simulink model "SVPWM_32bianhuan_"  (Simulink 7.6)
settings: Solver=ode45  StartTime=0.0  StopTime=0.5  FixedStep=1e-7  MaxStep=1e-5  MinStep=1e-6  RelTol=1e-3
libraries: powerlib x23, powerlib_extras x5, simulink x1
settings Model: Creator=Administrator  LastModifiedBy=huanglei
settings OptimizationCC: InitFltsAndDblsToZero=on
settings DebuggingCC: AlgebraicLoopMsg=none  SaveWithParameterizedLinksMsg=none  SignalResolutionControl=TryResolveAllWithWarning  MultiTaskDSMMsg=warning  MultiTaskCondExecSysMsg=none  StrictBusMsg=None
settings RTWCC: IncludeERTFirstTime=on
settings GRTTargetCC: TargetFcnLib=ansi_tfl_tmw.mat

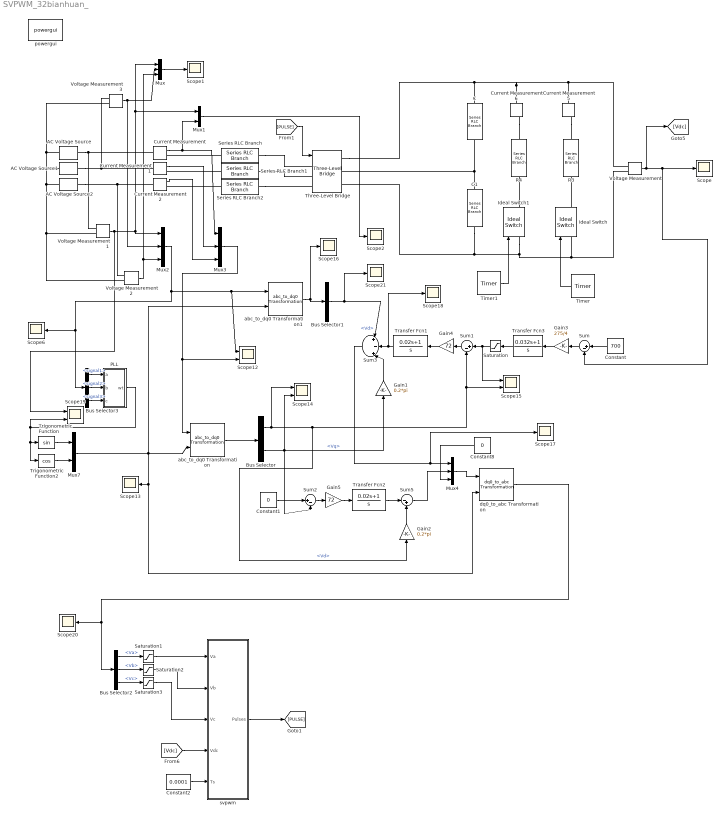
== system SVPWM_32bianhuan_ ==
  AC Voltage Source : powerlib/Electrical Sources/AC Voltage Source  DialogController=POWERSYS.PowerSysDialog  SystemSampleTime=-1  Amplitude=311  Phase=90  Frequency=50  SampleTime=0  Measurements=None
  AC Voltage Source1 : powerlib/Electrical Sources/AC Voltage Source  DialogController=POWERSYS.PowerSysDialog  SystemSampleTime=-1  Amplitude=311  Phase=-30  Frequency=50  SampleTime=0  Measurements=None
  AC Voltage Source2 : powerlib/Electrical Sources/AC Voltage Source  DialogController=POWERSYS.PowerSysDialog  SystemSampleTime=-1  Amplitude=311  Phase=210  Frequency=50  SampleTime=0  Measurements=None
  Bus Selector : BusSelector  OutputSignals=Vd,Vq
  Bus Selector1 : BusSelector  OutputSignals=Vd
  Bus Selector2 : BusSelector  OutputSignals=Va,Vb,Vc
  Bus Selector3 : BusSelector  OutputSignals=signal1,signal2,signal3
  C : powerlib/Elements/Series RLC Branch  DialogController=POWERSYS.PowerSysDialog  PhysicalDomain=powersysdomain  SubClassName=unknown  LeftPortType=p1  RightPortType=p1  LConnTagsString=__new0  RConnTagsString=__new0  BranchType=C  Resistance=1  Inductance=1e-3  SetiL0=off  InitialCurrent=0  Capacitance=1e-3  Setx0=off  InitialVoltage=0  Measurements=None
  C1 : powerlib/Elements/Series RLC Branch  DialogController=POWERSYS.PowerSysDialog  PhysicalDomain=powersysdomain  SubClassName=unknown  LeftPortType=p1  RightPortType=p1  LConnTagsString=__new0  RConnTagsString=__new0  BranchType=C  Resistance=1  Inductance=1e-3  SetiL0=off  InitialCurrent=0  Capacitance=1e-3  Setx0=off  InitialVoltage=0  Measurements=None
  Constant : Constant  Value=700
  Constant1 : Constant  Value=0
  Constant2 : Constant  Value=0.0001
  Constant8 : Constant  Value=0
  Current Measurement{,1..2,5..6} (5 alike) : powerlib/Measurements/Current Measurement  DialogController=POWERSYS.PowerSysDialog  SystemSampleTime=-1  PhasorSimulation=off  OutputType=Complex  PSBequivalent=0
  Gain1 : Gain  Gain=0.2*pi
  Gain2 : Gain  Gain=0.2*pi
  Gain3 : Gain  Gain=275/4
  Gain4 : Gain  Gain=72
  Gain5 : Gain  Gain=72
  Ideal Switch : powerlib/Power Electronics/Ideal Switch  DialogController=POWERSYS.PowerSysDialog  SystemSampleTime=-1  Ron=0.001  Lon=0  IC=0  Rs=1e5  Cs=inf  Measurements=on
  Ideal Switch1 : powerlib/Power Electronics/Ideal Switch  DialogController=POWERSYS.PowerSysDialog  SystemSampleTime=-1  Ron=0.001  Lon=0  IC=0  Rs=1e5  Cs=inf  Measurements=on
  Mux{,2..4} (4 alike) : Mux  Inputs=3
  Mux1 : Mux  Inputs=2
  Mux7 : Mux  Inputs=2
  PLL : Subsystem
  R3 : powerlib/Elements/Series RLC Branch  DialogController=POWERSYS.PowerSysDialog  PhysicalDomain=powersysdomain  SubClassName=unknown  LeftPortType=p1  RightPortType=p1  LConnTagsString=__new0  RConnTagsString=__new0  BranchType=R  Resistance=100  Inductance=1e-3  SetiL0=off  InitialCurrent=0  Capacitance=1e-6  Setx0=off  InitialVoltage=0  Measurements=None
  R4 : powerlib/Elements/Series RLC Branch  DialogController=POWERSYS.PowerSysDialog  PhysicalDomain=powersysdomain  SubClassName=unknown  LeftPortType=p1  RightPortType=p1  LConnTagsString=__new0  RConnTagsString=__new0  BranchType=R  Resistance=50  Inductance=1e-3  SetiL0=off  InitialCurrent=0  Capacitance=1e-6  Setx0=off  InitialVoltage=0  Measurements=None
  Saturation : Saturate  UpperLimit=200  LowerLimit=-200
  Saturation1 : Saturate  UpperLimit=220  LowerLimit=-220
  Saturation2 : Saturate  UpperLimit=220  LowerLimit=-220
  Saturation3 : Saturate  UpperLimit=220  LowerLimit=-220
  Scope{,1..2,6,13,16..18,20..21} (10 alike) : Scope
      Scope settings: TimeRange=0.5  YMin=698.5  YMax=707
      Scope1 settings: YMin=-400  YMax=400
      Scope13 settings: YMin=-1  YMax=0.6  SaveName=ScopeData13
      Scope16 settings: YMin=-25  YMax=325  SaveName=ScopeData16
      Scope17 settings: YMin=21050  YMax=22150  SaveName=ScopeData17
      Scope18 settings: YMin=-20775  YMax=-20425  SaveName=ScopeData18
      Scope2 settings: YMin=-350  YMax=350  SaveName=ScopeData2
      Scope20 settings: YMin=-1  YMax=1  SaveName=ScopeData20
      Scope21 settings: YMin=311  YMax=311  SaveName=ScopeData21
      Scope6 settings: YMin=-400  YMax=400  SaveName=ScopeData6
  Scope{12,14..15,19} (4 alike) : Scope  NumInputPorts=2
      Scope12 settings: YMin=-4~-5  YMax=4~5  SaveName=ScopeData12
      Scope14 settings: YMin=15~-2.25  YMax=26~3.25  SaveName=ScopeData14
      Scope15 settings: YMin=-503.7~-1  YMax=-503.425~1  SaveName=ScopeData15
      Scope19 settings: YMin=0~-5  YMax=6.5~5  SaveName=ScopeData19
  Series RLC Branch : powerlib/Elements/Series RLC Branch  DialogController=POWERSYS.PowerSysDialog  PhysicalDomain=powersysdomain  SubClassName=unknown  LeftPortType=p1  RightPortType=p1  LConnTagsString=__new0  RConnTagsString=__new0  BranchType=RL  Resistance=0.1  Inductance=2e-3  SetiL0=off  InitialCurrent=0  Capacitance=1e-6  Setx0=off  InitialVoltage=0  Measurements=None
  Series RLC Branch1 : powerlib/Elements/Series RLC Branch  DialogController=POWERSYS.PowerSysDialog  PhysicalDomain=powersysdomain  SubClassName=unknown  LeftPortType=p1  RightPortType=p1  LConnTagsString=__new0  RConnTagsString=__new0  BranchType=RL  Resistance=0.1  Inductance=2e-3  SetiL0=off  InitialCurrent=0  Capacitance=1e-6  Setx0=off  InitialVoltage=0  Measurements=None
  Series RLC Branch2 : powerlib/Elements/Series RLC Branch  DialogController=POWERSYS.PowerSysDialog  PhysicalDomain=powersysdomain  SubClassName=unknown  LeftPortType=p1  RightPortType=p1  LConnTagsString=__new0  RConnTagsString=__new0  BranchType=RL  Resistance=0.1  Inductance=2e-3  SetiL0=off  InitialCurrent=0  Capacitance=1e-6  Setx0=off  InitialVoltage=0  Measurements=None
  Sum : Sum  Inputs=|+-
  Sum1 : Sum  Inputs=|+-
  Sum2 : Sum  Inputs=|+-
  Sum3 : Sum  Inputs=|+|-|+|
  Sum5 : Sum  Inputs=|-+
  Three-Level Bridge : powerlib/Power Electronics/Three-Level Bridge  DialogController=POWERSYS.PowerSysDialog  SystemSampleTime=-1  Arms=3  SnubberResistance=1e5  SbubberCapacitance=inf  Device=IGBT / Diodes  Ron=1e-3  ForwardVoltages="[  0  0  ]"  Measurements=None
  Timer : powerlib_extras/Control  Blocks/Timer  DialogController=POWERSYS.PowerSysDialog  SystemSampleTime=-1  t=[0 0.3]  e=[0 1]
  Timer1 : powerlib_extras/Control  Blocks/Timer  DialogController=POWERSYS.PowerSysDialog  SystemSampleTime=-1  t=[0 0.3]  e=[1 0]
  Transfer Fcn1 : TransferFcn  Numerator=[0.02 1]  Denominator=[1 0]
  Transfer Fcn2 : TransferFcn  Numerator=[0.02 1]  Denominator=[1 0]
  Transfer Fcn3 : TransferFcn  Numerator=[0.032 1]  Denominator=[1 0]
  Trigonometric Function : Trigonometry
  Trigonometric Function2 : Trigonometry  Operator=cos
  Voltage Measurement{,1..3} (4 alike) : powerlib/Measurements/Voltage Measurement  DialogController=POWERSYS.PowerSysDialog  SystemSampleTime=-1  PhasorSimulation=off  OutputType=Complex  PSBequivalent=0
  abc_to_dq0 Transformation : powerlib_extras/Measurements/abc_to_dq0 Transformation  DialogController=POWERSYS.PowerSysDialog  SystemSampleTime=-1
  abc_to_dq0 Transformation1 : powerlib_extras/Measurements/abc_to_dq0 Transformation  DialogController=POWERSYS.PowerSysDialog  SystemSampleTime=-1
  dq0_to_abc Transformation : powerlib_extras/Measurements/dq0_to_abc Transformation  DialogController=POWERSYS.PowerSysDialog  SystemSampleTime=-1
  powergui : powerlib/powergui  Priority=1  SystemSampleTime=-1  SimulationMode=Discrete  SampleTime=50e-6  frequency=60  SPID=off  DisableSnubberDevices=off  DisableRonSwitches=off  DisableVfSwitches=off  SwTol=0  Interpol=off  frequencyindice=50  echomessages=off  HookPort=off  DisplayEquations=off  FunctionMessages=off  EnableUseOfTLC=off  x0status=blocks  RestoreLinks=warning  ResistiveCurrentMeasurement=off  Frange=[0:2:500]  Ylog=off  Xlog=on  ShowGrid=off  save=off  variable=ZData  ZoomFFT=off  StartTime=0.0  cycles=1  DisplayStyle=1  fundamental=60  FreqAxis=off  MaxFrequency=1000  frequencyindicesteady=1  RmsSteady=1  display=off  Ts=0  methode=off
  svpwm : Subsystem
  wires:
  Voltage Measurement/1 -> Scope/1, Sum/2, [Vdc]
  Current Measurement/1 -> Mux1/2, Mux3/1
  Voltage Measurement1/1 -> Scope19/1, Mux2/1, Mux/1, Mux1/1
  Voltage Measurement3/1 -> Mux/2, Mux2/2
  Mux/1 -> Scope1/1
  Mux1/1 -> Scope2/1
  Voltage Measurement2/1 -> Mux/3, Mux2/3
  Constant/1 -> Sum/1
  Mux2/1 -> Scope6/1, Bus Selector3/1, Scope12/1, abc_to_dq0 Transformation1/1
  Current Measurement1/1 -> Mux3/2
  Current Measurement2/1 -> Mux3/3
  Mux3/1 -> abc_to_dq0 Transformation/1, Scope12/2
  abc_to_dq0 Transformation/1 -> Bus Selector/1
  Bus Selector/1 -> Gain2/1, Sum1/2, Scope15/2, Scope14/1  "<Vd>"
  Sum1/1 -> Gain4/1
  Constant1/1 -> Sum2/1
  Bus Selector/2 -> Scope14/2, Gain1/1, Sum2/2  "<Vq>"
  Sum2/1 -> Gain5/1
  Gain1/1 -> Sum3/3
  Gain2/1 -> Sum5/2
  abc_to_dq0 Transformation1/1 -> Bus Selector1/1, Scope16/1
  Bus Selector1/1 -> Sum3/1, Scope21/1  "<Vd>"
  Sum3/1 -> Mux4/1, Scope17/1
  Sum5/1 -> Mux4/2
  Mux4/1 -> dq0_to_abc Transformation/1
  dq0_to_abc Transformation/1 -> Bus Selector2/1, Scope20/1
  Constant8/1 -> Mux4/3
  Trigonometric Function2/1 -> Mux7/2
  Trigonometric Function/1 -> Mux7/1
  Bus Selector3/1 -> PLL/1(a)  "<signal1>"
  Bus Selector3/2 -> PLL/2(b)  "<signal2>"
  Bus Selector3/3 -> PLL/3(c)  "<signal3>"
  Mux7/1 -> abc_to_dq0 Transformation1/2, abc_to_dq0 Transformation/2, Scope13/1, dq0_to_abc Transformation/2
  PLL/1(wt) -> Trigonometric Function/1, Trigonometric Function2/1, Scope19/2
  Sum/1 -> Gain3/1
  Gain3/1 -> Transfer Fcn3/1
  Gain4/1 -> Transfer Fcn1/1
  Gain5/1 -> Transfer Fcn2/1
  Transfer Fcn3/1 -> Saturation/1
  Transfer Fcn2/1 -> Sum5/1
  Transfer Fcn1/1 -> Sum3/2, Scope18/1
  Saturation/1 -> Scope15/1, Sum1/1
  Timer/1 -> Ideal Switch/1
  Timer1/1 -> Ideal Switch1/1
  Constant2/1 -> svpwm/5(Ts)
  [Vdc] -> svpwm/4(Vdc)
  svpwm/1(Pulses) -> [PULSE]
  [PULSE] -> Three-Level Bridge/1
  Bus Selector2/1 -> Saturation1/1  "<Va>"
  Saturation1/1 -> svpwm/1(Va)
  Bus Selector2/2 -> Saturation2/1  "<Vb>"
  Bus Selector2/3 -> Saturation3/1  "<Vc>"
  Saturation2/1 -> svpwm/2(Vb)
  Saturation3/1 -> svpwm/3(Vc)
  connections:
  AC Voltage Source/RConn1 -- Current Measurement/LConn1 -- Voltage Measurement1/LConn1
  AC Voltage Source1/RConn1 -- Current Measurement1/LConn1 -- Voltage Measurement3/LConn1
  AC Voltage Source2/RConn1 -- Current Measurement2/LConn1 -- Voltage Measurement2/LConn1
  Voltage Measurement3/LConn2 -- Voltage Measurement1/LConn2 -- Voltage Measurement2/LConn2 -- AC Voltage Source2/LConn1 -- AC Voltage Source1/LConn1 -- AC Voltage Source/LConn1
  Series RLC Branch/LConn1 -- Current Measurement/RConn1
  Series RLC Branch1/LConn1 -- Current Measurement1/RConn1
  Series RLC Branch2/LConn1 -- Current Measurement2/RConn1
  Current Measurement5/RConn1 -- R3/RConn1
  Ideal Switch/RConn1 -- R3/LConn1
  Current Measurement6/RConn1 -- R4/RConn1
  Ideal Switch1/RConn1 -- R4/LConn1
  Series RLC Branch/RConn1 -- Three-Level Bridge/LConn1
  Series RLC Branch1/RConn1 -- Three-Level Bridge/LConn2
  Series RLC Branch2/RConn1 -- Three-Level Bridge/LConn3
  C1/LConn1 -- C/RConn1 -- Three-Level Bridge/RConn2
  Three-Level Bridge/RConn1 -- C/LConn1 -- Current Measurement6/LConn1 -- Voltage Measurement/LConn1 -- Current Measurement5/LConn1
  C1/RConn1 -- Three-Level Bridge/RConn3 -- Ideal Switch1/LConn1 -- Voltage Measurement/LConn2 -- Ideal Switch/LConn1

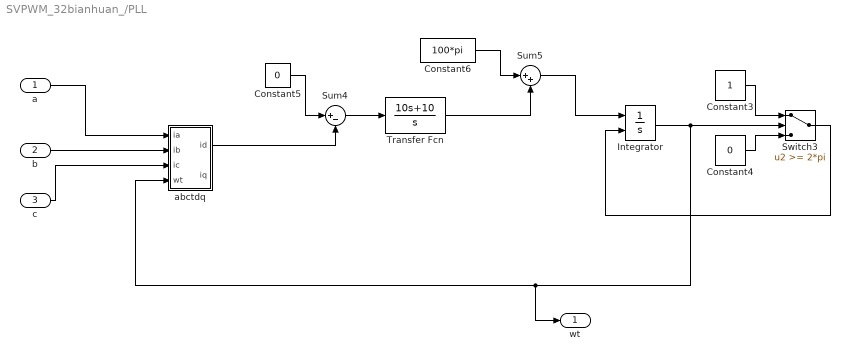
== system SVPWM_32bianhuan_/PLL ==
  a : Inport
  b : Inport  Port=2
  c : Inport  Port=3
  Constant3 : Constant
  Constant4 : Constant  Value=0
  Constant5 : Constant  Value=0
  Constant6 : Constant  Value=100*pi
  Integrator : Integrator  ExternalReset=rising
  Sum4 : Sum  Inputs=|+-
  Sum5 : Sum  Inputs=|++
  Switch3 : Switch  Threshold=2*pi
  Transfer Fcn : TransferFcn  Numerator=[10 10]  Denominator=[1 0]
  abctdq : Subsystem
  wt : Outport
  wires:
  Constant3/1 -> Switch3/1
  Switch3/1 -> Integrator/2
  Constant4/1 -> Switch3/3
  Integrator/1 -> Switch3/2, wt/1, abctdq/4(wt)
  a/1 -> abctdq/1(ia)
  Constant5/1 -> Sum4/1
  abctdq/1(id) -> Sum4/2
  b/1 -> abctdq/2(ib)
  c/1 -> abctdq/3(ic)
  Constant6/1 -> Sum5/1
  Sum5/1 -> Integrator/1
  Transfer Fcn/1 -> Sum5/2
  Sum4/1 -> Transfer Fcn/1

== system SVPWM_32bianhuan_/svpwm ==
  Va : Inport
  Vb : Inport  Port=2
  Vc : Inport  Port=3
  Vdc : Inport  Port=4
  Ts : Inport  Port=5
  Repeating Sequence1 : simulink/Sources/Repeating Sequence  SystemSampleTime=-1  rep_seq_t=[0 0.00005 0.0001]  rep_seq_y=[0 0.00005 0]
  Scope : Scope
      settings: SaveName=ScopeData7
  Sub4 abc__alpha_beta : Subsystem
  Subsystem5 : Subsystem
  Pulses : Outport
  wires:
  Vc/1 -> Sub4 abc__alpha_beta/3(Vc)
  Sub4 abc__alpha_beta/2(Vbeta) -> Subsystem5/2(Vbeta)
  Sub4 abc__alpha_beta/1(Valfa) -> Subsystem5/1(Valfa), Scope/1
  Vb/1 -> Sub4 abc__alpha_beta/2(Vb)
  Va/1 -> Sub4 abc__alpha_beta/1(Va)
  Subsystem5/1(Pulses) -> Pulses/1
  Vdc/1 -> Subsystem5/3(Vdc)
  Ts/1 -> Subsystem5/4(Ts)
  Repeating Sequence1/1 -> Subsystem5/5(wave)

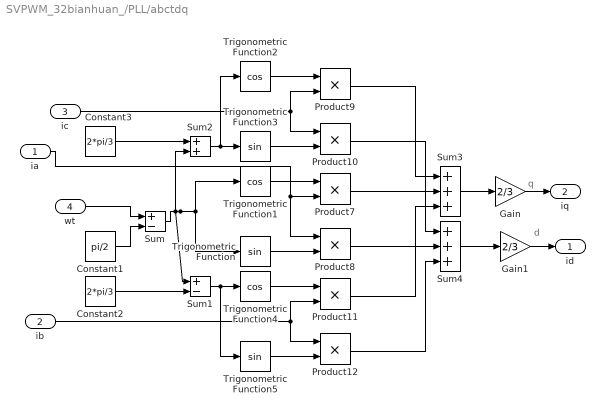
== system SVPWM_32bianhuan_/PLL/abctdq ==
  note: d
  note: q
  ia : Inport
  ib : Inport  Port=2
  ic : Inport  Port=3
  wt : Inport  Port=4
  Constant1 : Constant  Value=pi/2
  Constant2 : Constant  Value=2*pi/3
  Constant3 : Constant  Value=2*pi/3
  Gain : Gain  Gain=2/3
  Gain1 : Gain  Gain=2/3
  Product{7..12} (6 alike) : Product  RndMeth=Zero
  Sum : Sum  Inputs=+-
  Sum1 : Sum  Inputs=+-
  Sum2 : Sum
  Sum3 : Sum  Inputs=+++
  Sum4 : Sum  Inputs=+++
  Trigonometric Function : Trigonometry
  Trigonometric Function1 : Trigonometry  Operator=cos
  Trigonometric Function2 : Trigonometry  Operator=cos
  Trigonometric Function3 : Trigonometry
  Trigonometric Function4 : Trigonometry  Operator=cos
  Trigonometric Function5 : Trigonometry
  id : Outport
  iq : Outport  Port=2
  wires:
  ic/1 -> Product10/1, Product9/2
  ia/1 -> Product8/1, Product7/2
  ib/1 -> Product12/1, Product11/2
  Sum4/1 -> Gain1/1
  Sum3/1 -> Gain/1
  Product11/1 -> Sum3/3
  Product9/1 -> Sum3/1
  Product10/1 -> Sum4/1
  Product12/1 -> Sum4/3
  Product7/1 -> Sum3/2
  Product8/1 -> Sum4/2
  Trigonometric Function5/1 -> Product12/2
  Trigonometric Function4/1 -> Product11/1
  Trigonometric Function/1 -> Product8/2
  Trigonometric Function1/1 -> Product7/1
  Trigonometric Function3/1 -> Product10/2
  Trigonometric Function2/1 -> Product9/1
  Sum1/1 -> Trigonometric Function4/1, Trigonometric Function5/1
  Constant1/1 -> Sum/2
  Sum2/1 -> Trigonometric Function2/1, Trigonometric Function3/1
  Constant3/1 -> Sum2/1
  Constant2/1 -> Sum1/2
  Sum/1 -> Trigonometric Function/1, Trigonometric Function1/1, Sum1/1, Sum2/2
  wt/1 -> Sum/1
  Gain/1 -> iq/1
  Gain1/1 -> id/1

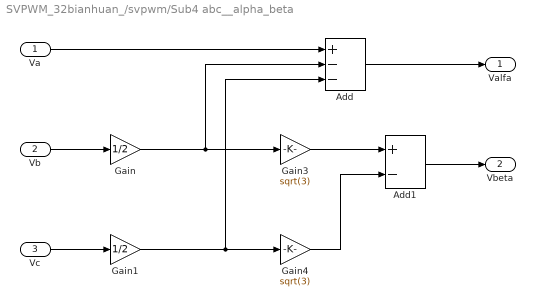
== system SVPWM_32bianhuan_/svpwm/Sub4 abc__alpha_beta ==
  Va : Inport
  Vb : Inport  Port=2
  Vc : Inport  Port=3
  Add : Sum  Inputs=+--
  Add1 : Sum  Inputs=+-
  Gain : Gain  Gain=1/2
  Gain1 : Gain  Gain=1/2
  Gain3 : Gain  Gain=sqrt(3)
  Gain4 : Gain  Gain=sqrt(3)
  Valfa : Outport
  Vbeta : Outport  Port=2
  wires:
  Vc/1 -> Gain1/1
  Vb/1 -> Gain/1
  Va/1 -> Add/1
  Add/1 -> Valfa/1
  Gain/1 -> Add/2, Gain3/1
  Gain1/1 -> Add/3, Gain4/1
  Gain3/1 -> Add1/1
  Gain4/1 -> Add1/2
  Add1/1 -> Vbeta/1

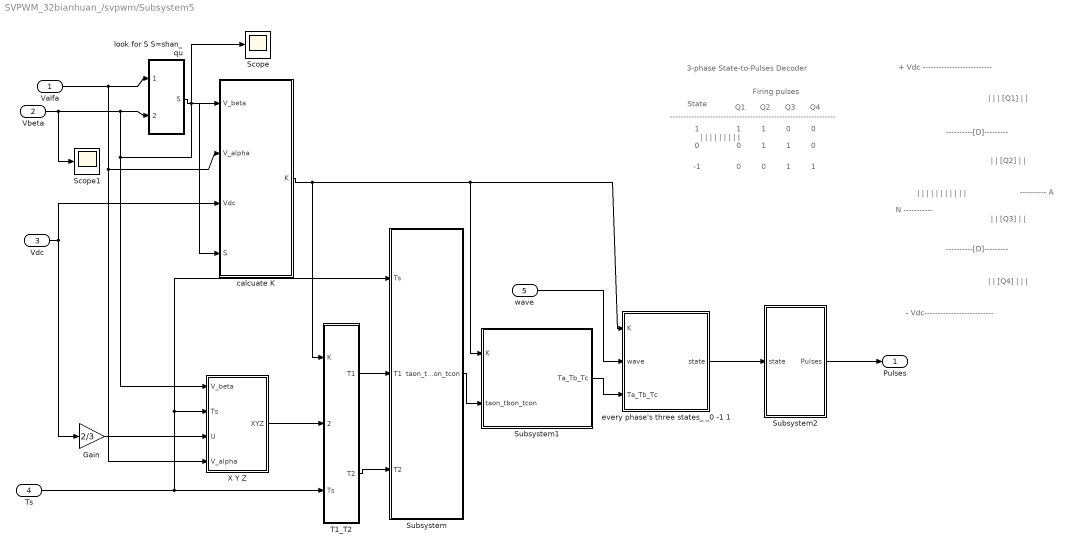
== system SVPWM_32bianhuan_/svpwm/Subsystem5 ==
  note: |
      | |
      | |
      | [Q1]
      | |
      | |
  note: |
      | |
      | [Q2]
      | |
      | |
  note: |
      | |
      | [Q3]
      | |
      | |
  note: |
      | |
      | [Q4]
      | |
      | |
      | |
  note: ----------[D]---------
  note: ----------[D]---------
  note: ---------- A
  note: |
      | |
      | |
      | |
      | |
      | |
      | |
      | |
      | |
      | |
      | |
  note: N -----------
  note: - Vdc--------------------------
  note: + Vdc --------------------------
  note: State
  note: 1
  note: Firing pulses
  note: 1
  note: 1
  note: 0
  note: 0
  note: Q1
  note: Q2
  note: Q3
  note: Q4
  note: 0
  note: 0
  note: 1
  note: 1
  note: 0
  note: -1
  note: 0
  note: 0
  note: 1
  note: 1
  note: |
      | |
      | |
      | |
      | |
      | |
      | |
      | |
      | |
  note: --------------------------------------------------------------
  note: 3-phase State-to-Pulses Decoder
  Valfa : Inport
  Vbeta : Inport  Port=2
  Vdc : Inport  Port=3
  Ts : Inport  Port=4
  wave : Inport  Port=5
  Gain : Gain  Gain=2/3
  Scope : Scope
      settings: SaveName=ScopeData4
  Scope1 : Scope
      settings: SaveName=ScopeData32
  Subsystem : Subsystem
  Subsystem1 : Subsystem
  Subsystem2 : Subsystem
  T1_T2 : Subsystem
  X Y Z : Subsystem
  calcuate K : Subsystem
  every phase's three states_ _0 -1 1 : Subsystem
  "look for S S=shan_qu    " : Subsystem
  Pulses : Outport
  wires:
  Valfa/1 -> "look for S S=shan_qu    "/1(Ualpha), X Y Z/4(V_alpha), calcuate K/2(V_alpha)
  Vbeta/1 -> "look for S S=shan_qu    "/2(Ubeta), X Y Z/1(V_beta), calcuate K/1(V_beta), Scope1/1
  "look for S S=shan_qu    "/1("S ") -> Scope/1, calcuate K/4(S)
  Gain/1 -> X Y Z/3(U)
  X Y Z/1(XYZ) -> T1_T2/2(XYZ)
  Ts/1 -> T1_T2/3(Ts), X Y Z/2(Ts), Subsystem/1(Ts)
  T1_T2/1(T1) -> Subsystem/2(T1)
  T1_T2/2(T2) -> Subsystem/3(T2)
  every phase's three states_ _0 -1 1/1(state) -> Subsystem2/1(state)
  Subsystem1/1(Ta_Tb_Tc) -> every phase's three states_ _0 -1 1/3(Ta_Tb_Tc)
  wave/1 -> every phase's three states_ _0 -1 1/2(wave)
  Subsystem2/1(Pulses) -> Pulses/1
  Vdc/1 -> Gain/1, calcuate K/3(Vdc)
  Subsystem/1(taon_tbon_tcon) -> Subsystem1/2(taon_tbon_tcon)
  calcuate K/1(K) -> T1_T2/1(K), Subsystem1/1(K), every phase's three states_ _0 -1 1/1(K)

== system SVPWM_32bianhuan_/svpwm/Subsystem5/Subsystem ==
  Ts : Inport
  T1 : Inport  Port=2
  T2 : Inport  Port=3
  Add1 : Sum
  Add2 : Sum
  Add4 : Sum  Inputs=+--
  Gain1 : Gain  Gain=1/4
  Gain2 : Gain  Gain=1/2
  Gain3 : Gain  Gain=1/2
  Mux : Mux  Inputs=3
  taon_tbon_tcon : Outport
  wires:
  T1/1 -> Gain2/1, Add4/2
  T2/1 -> Gain3/1, Add4/3
  Add4/1 -> Gain1/1
  Gain1/1 -> Add1/1, Mux/1
  Gain2/1 -> Add1/2
  Gain3/1 -> Add2/2
  Add1/1 -> Add2/1, Mux/2
  Ts/1 -> Add4/1
  Add2/1 -> Mux/3
  Mux/1 -> taon_tbon_tcon/1

== system SVPWM_32bianhuan_/svpwm/Subsystem5/Subsystem1 ==
  K : Inport
  taon_tbon_tcon : Inport  Port=2
  Demux : Demux  Outputs=3
  Mux1 : Mux  Inputs=3
  Ta : Subsystem
  Tb : Subsystem
  Tc : Subsystem
  Ta_Tb_Tc : Outport
  wires:
  Mux1/1 -> Ta_Tb_Tc/1
  Demux/3 -> Ta/3(tcon), Tb/3(tcon), Tc/3(tcon)
  Demux/2 -> Ta/2(tbon), Tb/2(tbon), Tc/2(tbon)
  Demux/1 -> Ta/1(taon), Tc/1(taon), Tb/1(taon)
  Tc/1(Tc) -> Mux1/3
  Tb/1(Tb) -> Mux1/2
  Ta/1(Ta) -> Mux1/1
  taon_tbon_tcon/1 -> Demux/1
  K/1 -> Ta/4(K), Tb/4(K), Tc/4(K)

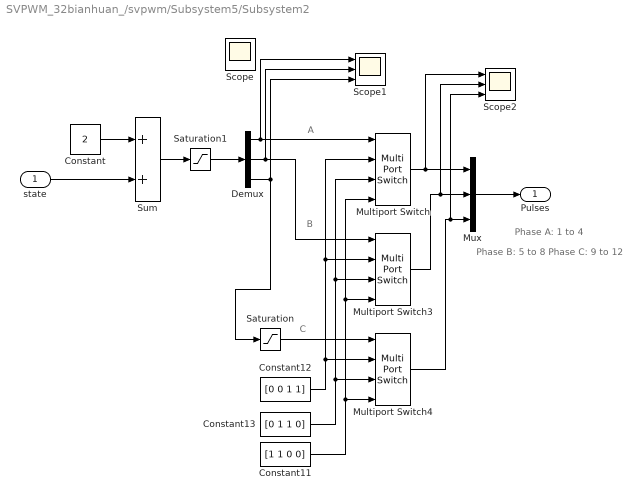
== system SVPWM_32bianhuan_/svpwm/Subsystem5/Subsystem2 ==
  note: Phase B: 5 to 8
      | Phase C: 9 to 12
  note: Phase A: 1 to 4
  note: A
  note: B
  note: C
  state : Inport
  Constant : Constant  Value=2
  Constant11 : Constant  Value=[1 1 0 0]
  Constant12 : Constant  Value=[0 0 1 1]
  Constant13 : Constant  Value=[0 1 1 0]
  Demux : Demux  Outputs=3
  Multiport Switch : MultiPortSwitch  zeroidx=off  InputSameDT=on
  Multiport Switch3 : MultiPortSwitch  zeroidx=off  InputSameDT=on
  Multiport Switch4 : MultiPortSwitch  zeroidx=off  InputSameDT=on
  Mux : Mux  Inputs=[4 4 4]
  Saturation : Saturate  UpperLimit=3  LowerLimit=1
  Saturation1 : Saturate  UpperLimit=1  LowerLimit=-1
  Scope : Scope
      settings: SaveName=ScopeData26
  Scope1 : Scope  NumInputPorts=3
      settings: YMin=-5~-5~-5  YMax=5~5~5  SaveName=ScopeData27
  Scope2 : Scope  NumInputPorts=3
      settings: YMin=0~0~-1  YMax=1~1~1  SaveName=ScopeData33
  Sum : Sum  SaturateOnIntegerOverflow=on  InputSameDT=on  OutDataTypeStr=Inherit: Same as first input
  Pulses : Outport
  wires:
  Mux/1 -> Pulses/1
  Demux/1 -> Multiport Switch/1, Scope1/1
  Demux/2 -> Multiport Switch3/1, Scope1/2
  Demux/3 -> Scope1/3, Saturation/1
  Constant12/1 -> Multiport Switch/2, Multiport Switch3/2, Multiport Switch4/2
  Constant13/1 -> Multiport Switch/3, Multiport Switch3/3, Multiport Switch4/3
  Constant11/1 -> Multiport Switch/4, Multiport Switch3/4, Multiport Switch4/4
  Multiport Switch/1 -> Mux/1, Scope2/1
  Multiport Switch3/1 -> Mux/2, Scope2/2
  Multiport Switch4/1 -> Mux/3, Scope2/3
  Constant/1 -> Sum/1
  state/1 -> Sum/2
  Saturation/1 -> Multiport Switch4/1
  Sum/1 -> Saturation1/1
  Saturation1/1 -> Demux/1

== system SVPWM_32bianhuan_/svpwm/Subsystem5/T1_T2 ==
  K : Inport
  XYZ : Inport  Port=2
  Ts : Inport  Port=3
  " calculate  T1" : Subsystem
  " calculate  T2" : Subsystem
  Demux : Demux  Outputs=3
  Demux1 : Demux  Outputs=3
  T1 : Outport
  T2 : Outport  Port=2
  wires:
  XYZ/1 -> Demux1/1, Demux/1
  K/1 -> " calculate  T2"/1(K), " calculate  T1"/1(K)
  Demux/1 -> " calculate  T1"/2(X)
  Demux/2 -> " calculate  T1"/3(Y)
  Demux/3 -> " calculate  T1"/4(Z)
  Demux1/1 -> " calculate  T2"/2(X)
  Demux1/2 -> " calculate  T2"/3(Y)
  Demux1/3 -> " calculate  T2"/4(Z)
  Ts/1 -> " calculate  T1"/5(Ts), " calculate  T2"/5(Ts)
  " calculate  T1"/1(T1) -> T1/1
  " calculate  T2"/1(T2) -> T2/1

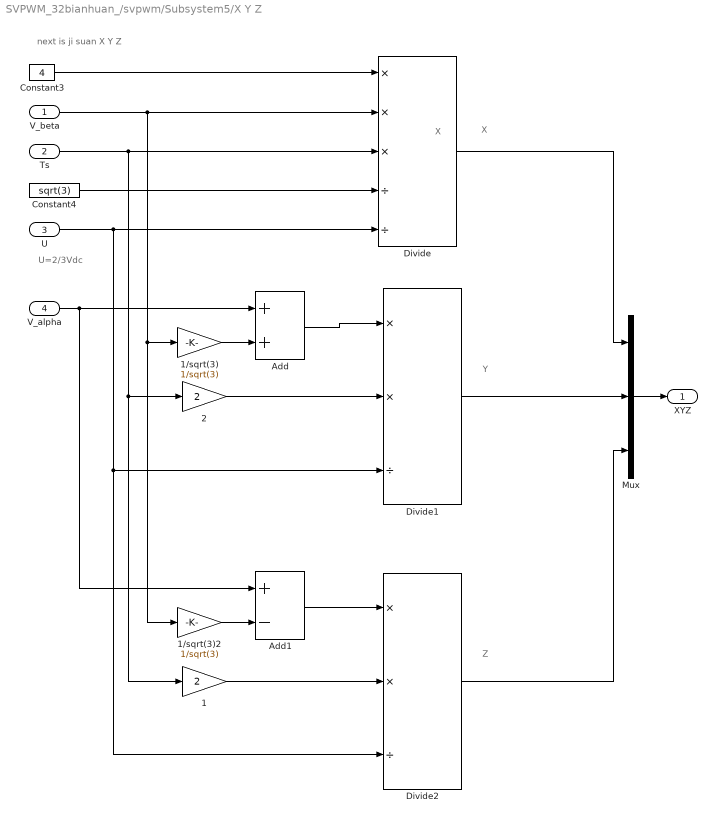
== system SVPWM_32bianhuan_/svpwm/Subsystem5/X Y Z ==
  note: next is ji suan X Y Z
  note: U=2/3Vdc
  note: X
  note: Y
  note: Z
  note: X
  V_beta : Inport
  Ts : Inport  Port=2
  U : Inport  Port=3
  V_alpha : Inport  Port=4
  1 : Gain  Gain=2
  1/sqrt(3) : Gain  Gain=1/sqrt(3)
  1/sqrt(3)2 : Gain  Gain=1/sqrt(3)
  2 : Gain  Gain=2
  Add : Sum
  Add1 : Sum  Inputs=+-
  Constant3 : Constant  Value=4
  Constant4 : Constant  Value=sqrt(3)
  Divide : Product  Inputs=***//
  Divide1 : Product  Inputs=**/
  Divide2 : Product  Inputs=**/
  Mux : Mux  Inputs=3
  XYZ : Outport
  wires:
  Constant3/1 -> Divide/1
  Ts/1 -> Divide/3, 2/1, 1/1
  Constant4/1 -> Divide/4
  U/1 -> Divide/5, Divide1/3, Divide2/3
  V_beta/1 -> Divide/2, 1/sqrt(3)/1, 1/sqrt(3)2/1
  V_alpha/1 -> Add/1, Add1/1
  1/sqrt(3)/1 -> Add/2
  2/1 -> Divide1/2
  Divide/1 -> Mux/1
  Divide1/1 -> Mux/2
  1/sqrt(3)2/1 -> Add1/2
  Add1/1 -> Divide2/1
  1/1 -> Divide2/2
  Divide2/1 -> Mux/3
  Mux/1 -> XYZ/1
  Add/1 -> Divide1/1

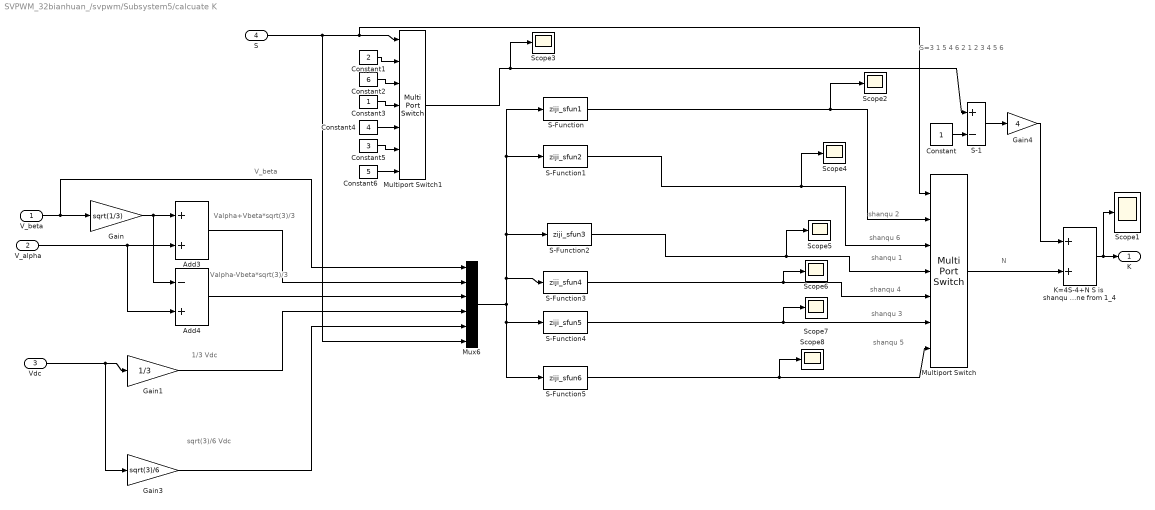
== system SVPWM_32bianhuan_/svpwm/Subsystem5/calcuate K ==
  note: N
  note: shanqu 6
  note: shanqu 5
  note: shanqu 4
  note: shanqu 3
  note: shanqu 2
  note: shanqu 1
  note: S=3    1    5    4    6    2
      |
      |      1    2    3    4    5    6
  note: V_beta
  note: Valpha+Vbeta*sqrt(3)/3
  note: Valpha-Vbeta*sqrt(3)/3
  note: 1/3 Vdc
  note: sqrt(3)/6 Vdc
  V_beta : Inport
  V_alpha : Inport  Port=2
  Vdc : Inport  Port=3
  S : Inport  Port=4
  Add3 : Sum
  Add4 : Sum  Inputs=-+
  Constant : Constant
  Constant1 : Constant  Value=2
  Constant2 : Constant  Value=6
  Constant3 : Constant
  Constant4 : Constant  Value=4
  Constant5 : Constant  Value=3
  Constant6 : Constant  Value=5
  Gain : Gain  Gain=sqrt(1/3)
  Gain1 : Gain  Gain=1/3
  Gain3 : Gain  Gain=sqrt(3)/6
  Gain4 : Gain  Gain=4
  K=4S-4+N S is  shanqu   N is zone from 1_4 : Sum
  Multiport Switch : MultiPortSwitch  Inputs=6  zeroidx=off
  Multiport Switch1 : MultiPortSwitch  Inputs=6  zeroidx=off
  Mux6 : Mux  Inputs=6
  S-1 : Sum  Inputs=+-
  S-Function : S-Function  FunctionName=ziji_sfun1  EnableBusSupport=off
  S-Function1 : S-Function  FunctionName=ziji_sfun2  EnableBusSupport=off
  S-Function2 : S-Function  FunctionName=ziji_sfun3  EnableBusSupport=off
  S-Function3 : S-Function  FunctionName=ziji_sfun4  EnableBusSupport=off
  S-Function4 : S-Function  FunctionName=ziji_sfun5  EnableBusSupport=off
  S-Function5 : S-Function  FunctionName=ziji_sfun6  EnableBusSupport=off
  Scope{1..8} (8 alike) : Scope
      Scope1 settings: SaveName=ScopeData6
      Scope2 settings: YMin=0  YMax=4  SaveName=ScopeData25
      Scope3 settings: YMin=1  SaveName=ScopeData5
      Scope4 settings: YMin=0  YMax=2  SaveName=ScopeData8
      Scope5 settings: YMin=0  YMax=4  SaveName=ScopeData9
      Scope6 settings: YMin=0  YMax=4  SaveName=ScopeData10
      Scope7 settings: YMin=0  YMax=4  SaveName=ScopeData11
      Scope8 settings: YMin=0  YMax=4  SaveName=ScopeData12
  K : Outport
  wires:
  V_alpha/1 -> Add3/2, Add4/2
  V_beta/1 -> Gain/1, Mux6/1
  Vdc/1 -> Gain1/1, Gain3/1
  Gain/1 -> Add3/1, Add4/1
  Gain4/1 -> K=4S-4+N S is  shanqu   N is zone from 1_4/1
  Multiport Switch/1 -> K=4S-4+N S is  shanqu   N is zone from 1_4/2
  Constant/1 -> S-1/2
  S-1/1 -> Gain4/1
  K=4S-4+N S is  shanqu   N is zone from 1_4/1 -> K/1, Scope1/1
  Add3/1 -> Mux6/2
  Add4/1 -> Mux6/3
  Gain1/1 -> Mux6/4
  Gain3/1 -> Mux6/5
  S/1 -> Mux6/6, Multiport Switch1/1, Multiport Switch/1
  Mux6/1 -> S-Function/1, S-Function1/1, S-Function2/1, S-Function3/1, S-Function4/1, S-Function5/1
  S-Function/1 -> Multiport Switch/2, Scope2/1
  S-Function1/1 -> Multiport Switch/3, Scope4/1
  S-Function2/1 -> Multiport Switch/4, Scope5/1
  S-Function3/1 -> Multiport Switch/5, Scope6/1
  S-Function4/1 -> Multiport Switch/6, Scope7/1
  S-Function5/1 -> Multiport Switch/7, Scope8/1
  Constant1/1 -> Multiport Switch1/2
  Constant2/1 -> Multiport Switch1/3
  Constant3/1 -> Multiport Switch1/4
  Constant4/1 -> Multiport Switch1/5
  Constant5/1 -> Multiport Switch1/6
  Constant6/1 -> Multiport Switch1/7
  Multiport Switch1/1 -> S-1/1, Scope3/1

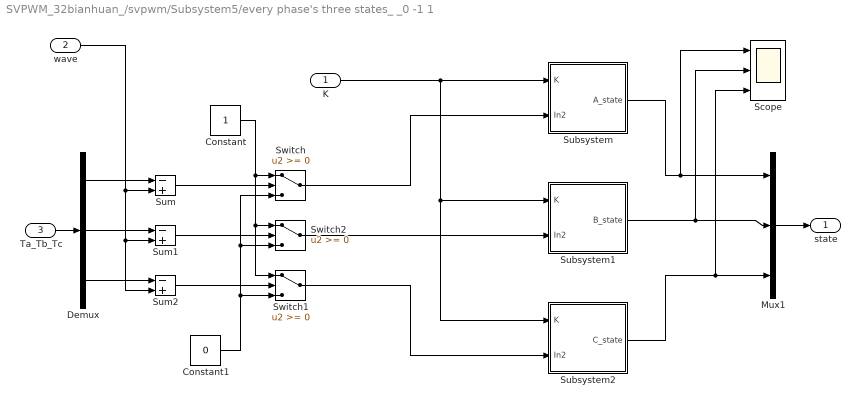
== system SVPWM_32bianhuan_/svpwm/Subsystem5/every phase's three states_ _0 -1 1 ==
  K : Inport
  wave : Inport  Port=2
  Ta_Tb_Tc : Inport  Port=3
  Constant : Constant
  Constant1 : Constant  Value=0
  Demux : Demux  Outputs=3
  Mux1 : Mux  Inputs=3
  Scope : Scope  NumInputPorts=3
      settings: YMin=-5~-5~-5  YMax=5~5~5  SaveName=ScopeData28
  Subsystem : Subsystem
  Subsystem1 : Subsystem
  Subsystem2 : Subsystem
  Sum : Sum  Inputs=-+  SaturateOnIntegerOverflow=on
  Sum1 : Sum  Inputs=-+  SaturateOnIntegerOverflow=on
  Sum2 : Sum  Inputs=-+  SaturateOnIntegerOverflow=on
  Switch : Switch  SaturateOnIntegerOverflow=on
  Switch1 : Switch  SaturateOnIntegerOverflow=on
  Switch2 : Switch  SaturateOnIntegerOverflow=on
  state : Outport
  wires:
  Switch1/1 -> Subsystem2/2(In2)
  Switch2/1 -> Subsystem1/2(In2)
  Constant1/1 -> Switch1/3, Switch2/3, Switch/3
  Constant/1 -> Switch/1, Switch2/1, Switch1/1
  Sum2/1 -> Switch1/2
  Sum1/1 -> Switch2/2
  Sum/1 -> Switch/2
  Demux/3 -> Sum2/1
  Demux/2 -> Sum1/1
  Demux/1 -> Sum/1
  wave/1 -> Sum1/2, Sum2/2, Sum/2
  Ta_Tb_Tc/1 -> Demux/1
  K/1 -> Subsystem/1(K), Subsystem1/1(K), Subsystem2/1(K)
  Switch/1 -> Subsystem/2(In2)
  Subsystem1/1(B_state) -> Mux1/2, Scope/2
  Subsystem/1(A_state) -> Mux1/1, Scope/1
  Subsystem2/1(C_state) -> Mux1/3, Scope/3
  Mux1/1 -> state/1

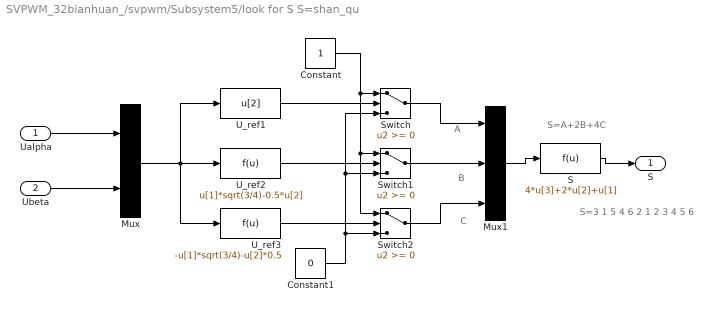
== system SVPWM_32bianhuan_/svpwm/Subsystem5/look for S S=shan_qu     ==
  note: A
  note: B
  note: C
  note: S=A+2B+4C
  note: S=3    1    5    4    6    2
      |
      |      1    2    3    4    5    6
  Ualpha : Inport
  Ubeta : Inport  Port=2
  Constant : Constant
  Constant1 : Constant  Value=0
  Mux : Mux  Inputs=2
  Mux1 : Mux  Inputs=3
  S : Fcn  Expr=4*u[3]+2*u[2]+u[1]
  Switch : Switch
  Switch1 : Switch
  Switch2 : Switch
  U_ref1 : Fcn  Expr=u[2]
  U_ref2 : Fcn  Expr=u[1]*sqrt(3/4)-0.5*u[2]
  U_ref3 : Fcn  Expr=-u[1]*sqrt(3/4)-u[2]*0.5
  "S " : Outport
  wires:
  Switch2/1 -> Mux1/3
  Switch/1 -> Mux1/1
  Ualpha/1 -> Mux/1
  Ubeta/1 -> Mux/2
  Mux/1 -> U_ref2/1, U_ref1/1, U_ref3/1
  U_ref1/1 -> Switch/2
  U_ref2/1 -> Switch1/2
  U_ref3/1 -> Switch2/2
  Constant/1 -> Switch/1, Switch2/1, Switch1/1
  Constant1/1 -> Switch/3, Switch1/3, Switch2/3
  Switch1/1 -> Mux1/2
  Mux1/1 -> S/1
  S/1 -> "S "/1

== system SVPWM_32bianhuan_/svpwm/Subsystem5/Subsystem1/Ta ==
  taon : Inport
  tbon : Inport  Port=2
  tcon : Inport  Port=3
  K : Inport  Port=4
  phaseA  qiehuan   dian Ta : MultiPortSwitch  Inputs=24  zeroidx=off
  Ta : Outport
  wires:
  phaseA  qiehuan   dian Ta/1 -> Ta/1
  tcon/1 -> phaseA  qiehuan   dian Ta/2, phaseA  qiehuan   dian Ta/6, phaseA  qiehuan   dian Ta/8, phaseA  qiehuan   dian Ta/11, phaseA  qiehuan   dian Ta/12, phaseA  qiehuan   dian Ta/13, phaseA  qiehuan   dian Ta/15, phaseA  qiehuan   dian Ta/17
  taon/1 -> phaseA  qiehuan   dian Ta/3, phaseA  qiehuan   dian Ta/5, phaseA  qiehuan   dian Ta/14, phaseA  qiehuan   dian Ta/18, phaseA  qiehuan   dian Ta/20, phaseA  qiehuan   dian Ta/23, phaseA  qiehuan   dian Ta/24, phaseA  qiehuan   dian Ta/25
  tbon/1 -> phaseA  qiehuan   dian Ta/4, phaseA  qiehuan   dian Ta/7, phaseA  qiehuan   dian Ta/9, phaseA  qiehuan   dian Ta/10, phaseA  qiehuan   dian Ta/16, phaseA  qiehuan   dian Ta/19, phaseA  qiehuan   dian Ta/21, phaseA  qiehuan   dian Ta/22
  K/1 -> phaseA  qiehuan   dian Ta/1

== system SVPWM_32bianhuan_/svpwm/Subsystem5/Subsystem1/Tb ==
  taon : Inport
  tbon : Inport  Port=2
  tcon : Inport  Port=3
  K : Inport  Port=4
  phaseA  qiehuan   dian Tb : MultiPortSwitch  Inputs=24  zeroidx=off
  Tb : Outport
  wires:
  phaseA  qiehuan   dian Tb/1 -> Tb/1
  taon/1 -> phaseA  qiehuan   dian Tb/2, phaseA  qiehuan   dian Tb/4, phaseA  qiehuan   dian Tb/7, phaseA  qiehuan   dian Tb/8, phaseA  qiehuan   dian Tb/9, phaseA  qiehuan   dian Tb/11, phaseA  qiehuan   dian Tb/13, phaseA  qiehuan   dian Tb/22
  tbon/1 -> phaseA  qiehuan   dian Tb/3, phaseA  qiehuan   dian Tb/5, phaseA  qiehuan   dian Tb/6, phaseA  qiehuan   dian Tb/12, phaseA  qiehuan   dian Tb/15, phaseA  qiehuan   dian Tb/17, phaseA  qiehuan   dian Tb/18, phaseA  qiehuan   dian Tb/24
  tcon/1 -> phaseA  qiehuan   dian Tb/10, phaseA  qiehuan   dian Tb/14, phaseA  qiehuan   dian Tb/16, phaseA  qiehuan   dian Tb/19, phaseA  qiehuan   dian Tb/20, phaseA  qiehuan   dian Tb/21, phaseA  qiehuan   dian Tb/23, phaseA  qiehuan   dian Tb/25
  K/1 -> phaseA  qiehuan   dian Tb/1

== system SVPWM_32bianhuan_/svpwm/Subsystem5/Subsystem1/Tc ==
  taon : Inport
  tbon : Inport  Port=2
  tcon : Inport  Port=3
  K : Inport  Port=4
  phaseA  qiehuan   dian Tc : MultiPortSwitch  Inputs=24  zeroidx=off
  Tc : Outport
  wires:
  phaseA  qiehuan   dian Tc/1 -> Tc/1
  tbon/1 -> phaseA  qiehuan   dian Tc/2, phaseA  qiehuan   dian Tc/8, phaseA  qiehuan   dian Tc/11, phaseA  qiehuan   dian Tc/13, phaseA  qiehuan   dian Tc/14, phaseA  qiehuan   dian Tc/20, phaseA  qiehuan   dian Tc/23, phaseA  qiehuan   dian Tc/25
  tcon/1 -> phaseA  qiehuan   dian Tc/3, phaseA  qiehuan   dian Tc/4, phaseA  qiehuan   dian Tc/5, phaseA  qiehuan   dian Tc/7, phaseA  qiehuan   dian Tc/9, phaseA  qiehuan   dian Tc/18, phaseA  qiehuan   dian Tc/22, phaseA  qiehuan   dian Tc/24
  taon/1 -> phaseA  qiehuan   dian Tc/6, phaseA  qiehuan   dian Tc/10, phaseA  qiehuan   dian Tc/12, phaseA  qiehuan   dian Tc/15, phaseA  qiehuan   dian Tc/16, phaseA  qiehuan   dian Tc/17, phaseA  qiehuan   dian Tc/19, phaseA  qiehuan   dian Tc/21
  K/1 -> phaseA  qiehuan   dian Tc/1

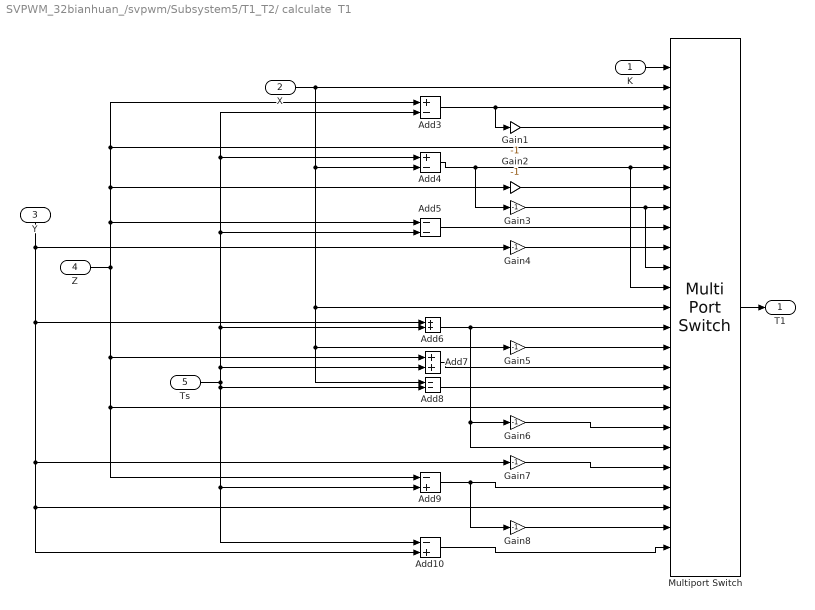
== system SVPWM_32bianhuan_/svpwm/Subsystem5/T1_T2/ calculate  T1 ==
  K : Inport
  X : Inport  Port=2
  Y : Inport  Port=3
  Z : Inport  Port=4
  Ts : Inport  Port=5
  Add10 : Sum  Inputs=-+
  Add3 : Sum  Inputs=+-
  Add4 : Sum  Inputs=+-
  Add5 : Sum  Inputs=--
  Add6 : Sum
  Add7 : Sum
  Add8 : Sum  Inputs=--
  Add9 : Sum  Inputs=-+
  Gain{1..8} (8 alike) : Gain  Gain=-1
  Multiport Switch : MultiPortSwitch  Inputs=24  zeroidx=off
  T1 : Outport
  wires:
  X/1 -> Add8/1, Gain5/1, Multiport Switch/13, Add4/2, Multiport Switch/2
  Z/1 -> Add9/1, Multiport Switch/18, Add7/1, Add5/1, Gain2/1, Multiport Switch/5, Add3/1
  Add3/1 -> Multiport Switch/3, Gain1/1
  Gain1/1 -> Multiport Switch/4
  Add4/1 -> Gain3/1, Multiport Switch/6, Multiport Switch/12
  Gain2/1 -> Multiport Switch/7
  Gain3/1 -> Multiport Switch/8, Multiport Switch/11
  Add5/1 -> Multiport Switch/9
  Y/1 -> Add10/2, Multiport Switch/23, Gain7/1, Add6/1, Gain4/1
  Gain4/1 -> Multiport Switch/10
  Add6/1 -> Multiport Switch/14, Gain6/1, Multiport Switch/20
  Gain5/1 -> Multiport Switch/15
  Add7/1 -> Multiport Switch/16
  Add8/1 -> Multiport Switch/17
  Gain6/1 -> Multiport Switch/19
  Gain7/1 -> Multiport Switch/21
  Add9/1 -> Multiport Switch/22, Gain8/1
  Gain8/1 -> Multiport Switch/24
  Add10/1 -> Multiport Switch/25
  Ts/1 -> Add3/2, Add4/1, Add5/2, Add6/2, Add7/2, Add8/2, Add9/2, Add10/1
  K/1 -> Multiport Switch/1
  Multiport Switch/1 -> T1/1

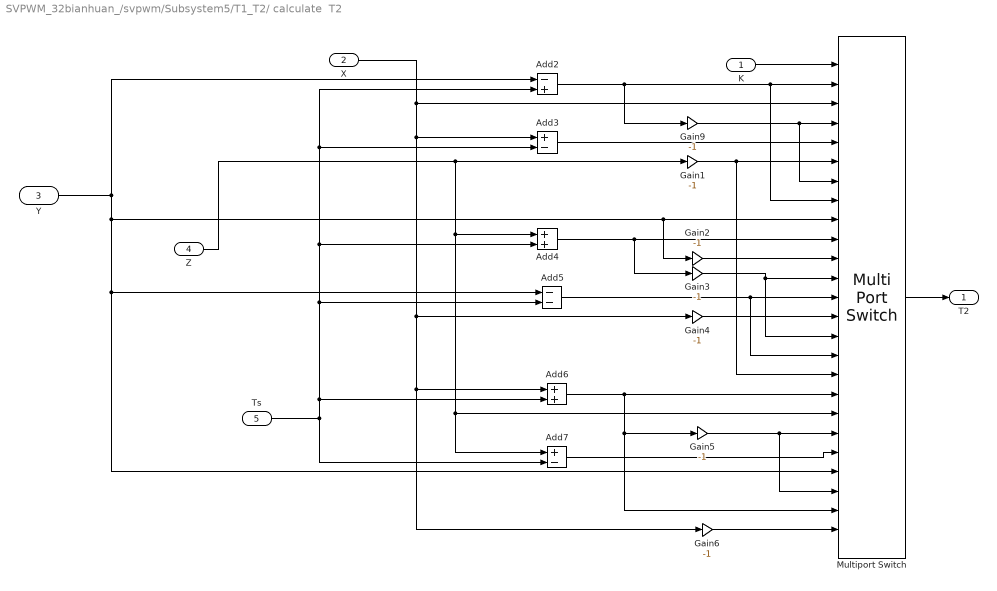
== system SVPWM_32bianhuan_/svpwm/Subsystem5/T1_T2/ calculate  T2 ==
  K : Inport
  X : Inport  Port=2
  Y : Inport  Port=3
  Z : Inport  Port=4
  Ts : Inport  Port=5
  Add2 : Sum  Inputs=-+
  Add3 : Sum  Inputs=+-
  Add4 : Sum
  Add5 : Sum  Inputs=--
  Add6 : Sum
  Add7 : Sum  Inputs=+-
  Gain{1..6,9} (7 alike) : Gain  Gain=-1
  Multiport Switch : MultiPortSwitch  Inputs=24  zeroidx=off
  T2 : Outport
  wires:
  Multiport Switch/1 -> T2/1
  K/1 -> Multiport Switch/1
  Ts/1 -> Add2/2, Add3/2, Add4/2, Add5/2, Add6/2, Add7/2
  Y/1 -> Add2/1, Multiport Switch/9, Gain2/1, Add5/1, Multiport Switch/22
  Add2/1 -> Gain9/1, Multiport Switch/2, Multiport Switch/8
  X/1 -> Multiport Switch/3, Add3/1, Gain4/1, Add6/1, Gain6/1
  Gain9/1 -> Multiport Switch/4, Multiport Switch/7
  Add3/1 -> Multiport Switch/5
  Z/1 -> Gain1/1, Add4/1, Multiport Switch/19, Add7/1
  Gain1/1 -> Multiport Switch/6, Multiport Switch/17
  Add4/1 -> Multiport Switch/10, Gain3/1
  Gain2/1 -> Multiport Switch/11
  Gain3/1 -> Multiport Switch/12, Multiport Switch/15
  Add5/1 -> Multiport Switch/13, Multiport Switch/16
  Gain4/1 -> Multiport Switch/14
  Add6/1 -> Multiport Switch/18, Gain5/1, Multiport Switch/24
  Gain5/1 -> Multiport Switch/20, Multiport Switch/23
  Add7/1 -> Multiport Switch/21
  Gain6/1 -> Multiport Switch/25

== system SVPWM_32bianhuan_/svpwm/Subsystem5/every phase's three states_ _0 -1 1/Subsystem ==
  K : Inport
  In2 : Inport  Port=2
  Constant2 : Constant
  Sum3 : Sum  Inputs=-+  SaturateOnIntegerOverflow=on
  pha qiehuan   dian Ta : MultiPortSwitch  Inputs=24  zeroidx=off
  A_state : Outport
  wires:
  In2/1 -> pha qiehuan   dian Ta/24, pha qiehuan   dian Ta/23, pha qiehuan   dian Ta/22, pha qiehuan   dian Ta/21, pha qiehuan   dian Ta/25, pha qiehuan   dian Ta/4, pha qiehuan   dian Ta/5, pha qiehuan   dian Ta/6, pha qiehuan   dian Ta/7, pha qiehuan   dian Ta/8, pha qiehuan   dian Ta/3, pha qiehuan   dian Ta/2, Sum3/2
  Constant2/1 -> Sum3/1
  Sum3/1 -> pha qiehuan   dian Ta/9, pha qiehuan   dian Ta/10, pha qiehuan   dian Ta/20, pha qiehuan   dian Ta/19, pha qiehuan   dian Ta/18, pha qiehuan   dian Ta/17, pha qiehuan   dian Ta/16, pha qiehuan   dian Ta/15, pha qiehuan   dian Ta/14, pha qiehuan   dian Ta/13, pha qiehuan   dian Ta/12, pha qiehuan   dian Ta/11
  K/1 -> pha qiehuan   dian Ta/1
  pha qiehuan   dian Ta/1 -> A_state/1

== system SVPWM_32bianhuan_/svpwm/Subsystem5/every phase's three states_ _0 -1 1/Subsystem1 ==
  K : Inport
  In2 : Inport  Port=2
  Constant2 : Constant
  Sum3 : Sum  Inputs=-+  SaturateOnIntegerOverflow=on
  "phaseA  qiehuan   dian " : MultiPortSwitch  Inputs=24  zeroidx=off
  B_state : Outport
  wires:
  In2/1 -> Sum3/2, "phaseA  qiehuan   dian "/5, "phaseA  qiehuan   dian "/6, "phaseA  qiehuan   dian "/7, "phaseA  qiehuan   dian "/8, "phaseA  qiehuan   dian "/9, "phaseA  qiehuan   dian "/10, "phaseA  qiehuan   dian "/11, "phaseA  qiehuan   dian "/16, "phaseA  qiehuan   dian "/15, "phaseA  qiehuan   dian "/14, "phaseA  qiehuan   dian "/13, "phaseA  qiehuan   dian "/12
  Constant2/1 -> Sum3/1
  K/1 -> "phaseA  qiehuan   dian "/1
  "phaseA  qiehuan   dian "/1 -> B_state/1
  Sum3/1 -> "phaseA  qiehuan   dian "/2, "phaseA  qiehuan   dian "/3, "phaseA  qiehuan   dian "/4, "phaseA  qiehuan   dian "/25, "phaseA  qiehuan   dian "/24, "phaseA  qiehuan   dian "/23, "phaseA  qiehuan   dian "/22, "phaseA  qiehuan   dian "/21, "phaseA  qiehuan   dian "/20, "phaseA  qiehuan   dian "/19, "phaseA  qiehuan   dian "/18, "phaseA  qiehuan   dian "/17

== system SVPWM_32bianhuan_/svpwm/Subsystem5/every phase's three states_ _0 -1 1/Subsystem2 ==
  K : Inport
  In2 : Inport  Port=2
  Constant2 : Constant
  Sum3 : Sum  Inputs=-+  SaturateOnIntegerOverflow=on
  "phaseA  qiehuan   dian " : MultiPortSwitch  Inputs=24  zeroidx=off
  C_state : Outport
  wires:
  Sum3/1 -> "phaseA  qiehuan   dian "/4, "phaseA  qiehuan   dian "/3, "phaseA  qiehuan   dian "/2, "phaseA  qiehuan   dian "/5, "phaseA  qiehuan   dian "/6, "phaseA  qiehuan   dian "/7, "phaseA  qiehuan   dian "/8, "phaseA  qiehuan   dian "/9, "phaseA  qiehuan   dian "/10, "phaseA  qiehuan   dian "/11, "phaseA  qiehuan   dian "/12, "phaseA  qiehuan   dian "/25
  "phaseA  qiehuan   dian "/1 -> C_state/1
  K/1 -> "phaseA  qiehuan   dian "/1
  Constant2/1 -> Sum3/1
  In2/1 -> Sum3/2, "phaseA  qiehuan   dian "/13, "phaseA  qiehuan   dian "/14, "phaseA  qiehuan   dian "/15, "phaseA  qiehuan   dian "/16, "phaseA  qiehuan   dian "/17, "phaseA  qiehuan   dian "/18, "phaseA  qiehuan   dian "/19, "phaseA  qiehuan   dian "/20, "phaseA  qiehuan   dian "/21, "phaseA  qiehuan   dian "/22, "phaseA  qiehuan   dian "/24, "phaseA  qiehuan   dian "/23
